simulink model "Hinf_sym1"  (R2023a)
settings: Solver=VariableStepAuto  StartTime=0.0  StopTime=500  RelTol=1e-3
InitFcn:
  | %Hinf_init
values from neighbouring files (symbols this model uses):
  C = [1 0 0 0; 0 1 0 0]    [Hinf_1DOF.m]    (also in Hinf_2DOFinit.m; Hinf_U_init.m; Hinf_WU_init.m; Hinf_init.m)
  dtheta_0 = 0    [Hinf_1DOF.m]    (also in Hinf_2DOFinit.m; Hinf_U_init.m; Hinf_WU_init.m; Hinf_init.m)
  dz_0 = 0    [Hinf_1DOF.m]    (also in Hinf_2DOFinit.m; Hinf_U_init.m; Hinf_WU_init.m; Hinf_init.m)
  fa_w = 0    [Hinf_1DOF.m]    (also in Hinf_2DOFinit.m; Hinf_U_init.m; Hinf_WU_init.m; Hinf_init.m)
  fm_w = s_param.g*s_param.m    [Hinf_1DOF.m]    (also in Hinf_2DOFinit.m; Hinf_U_init.m; Hinf_WU_init.m; Hinf_init.m)
  K = tf(ss(K.A,K.B,K.C,K.D))    [Hinf_U_init.m]    (also in Hinf_WU_init.m; Hinf_init.m)
  Km1 = 1.1    [Hinf_1DOF.m]    (also in Hinf_2DOFinit.m; Hinf_U_init.m; Hinf_WU_init.m; Hinf_init.m)
  Km1_real = Km1 + std_dev_Km*randn(1,1)    [Hinf_1DOF.m]    (also in Hinf_2DOFinit.m; Hinf_U_init.m; Hinf_WU_init.m; Hinf_init.m)
  Km2 = 1.1    [Hinf_1DOF.m]    (also in Hinf_2DOFinit.m; Hinf_U_init.m; Hinf_WU_init.m; Hinf_init.m)
  Km2_real = Km2 + std_dev_Km*randn(1,1)    [Hinf_1DOF.m]    (also in Hinf_2DOFinit.m; Hinf_U_init.m; Hinf_WU_init.m; Hinf_init.m)
  Kss = K    [Hinf_U_init.m]    (also in Hinf_WU_init.m; Hinf_init.m)
  out_rate = 0.001    [Hinf_1DOF.m]    (also in Hinf_2DOFinit.m; Hinf_U_init.m; Hinf_WU_init.m; Hinf_init.m)
  ss_global = ss(G)    [Hinf_init.m]
  T1 = 0.05    [Hinf_1DOF.m]    (also in Hinf_2DOFinit.m; Hinf_U_init.m; Hinf_WU_init.m; Hinf_init.m)
  T1_real = T1 + std_dev_T*randn(1,1)    [Hinf_1DOF.m]    (also in Hinf_2DOFinit.m; Hinf_U_init.m; Hinf_WU_init.m; Hinf_init.m)
  T2 = 0.15    [Hinf_1DOF.m]    (also in Hinf_2DOFinit.m; Hinf_U_init.m; Hinf_WU_init.m; Hinf_init.m)
  T2_real = T2 + std_dev_T*randn(1,1)    [Hinf_1DOF.m]    (also in Hinf_2DOFinit.m; Hinf_U_init.m; Hinf_WU_init.m; Hinf_init.m)
  theta_0_real = theta_0 + std_dev.theta_0*randn(1,1)    [Hinf_1DOF.m]    (also in Hinf_2DOFinit.m = theta_0+std_dev.theta_0*randn(1,1); Hinf_U_init.m = theta_0+std_dev.theta_0*randn(1,1); Hinf_WU_init.m = theta_0+std_dev.theta_0*randn(1,1); Hinf_init.m = theta_0+std_dev.theta_0*randn(1,1))
  theta_w = 0    [Hinf_1DOF.m]    (also in Hinf_2DOFinit.m; Hinf_U_init.m; Hinf_WU_init.m; Hinf_init.m)
  Tm1 = 1    [Hinf_1DOF.m]    (also in Hinf_2DOFinit.m; Hinf_U_init.m; Hinf_WU_init.m; Hinf_init.m)
  Tm1_real = Tm1 + std_dev_Tm*randn(1,1)    [Hinf_1DOF.m]    (also in Hinf_2DOFinit.m; Hinf_U_init.m; Hinf_WU_init.m; Hinf_init.m)
  Tm2 = 1    [Hinf_1DOF.m]    (also in Hinf_2DOFinit.m; Hinf_U_init.m; Hinf_WU_init.m; Hinf_init.m)
  Tm2_real = Tm2 + std_dev_Tm*randn(1,1)    [Hinf_1DOF.m]    (also in Hinf_2DOFinit.m; Hinf_U_init.m; Hinf_WU_init.m; Hinf_init.m)
  z_0_real = z_0 + std_dev.z_0*randn(1,1)    [Hinf_1DOF.m]    (also in Hinf_2DOFinit.m = z_0+std_dev.z_0*randn(1,1); Hinf_U_init.m = z_0+std_dev.z_0*randn(1,1); Hinf_WU_init.m = z_0+std_dev.z_0*randn(1,1); Hinf_init.m = z_0+std_dev.z_0*randn(1,1))
  z_w = 200    [Hinf_1DOF.m]    (also in Hinf_2DOFinit.m = 400; Hinf_U_init.m = 400; Hinf_WU_init.m = 400; Hinf_init.m = 400)
undefined symbols (not defined in the file or in its folder): s_param, s_param_r, std_dev
libraries: simulink x8
settings Model: Creator=franc  LastModifiedBy=franc

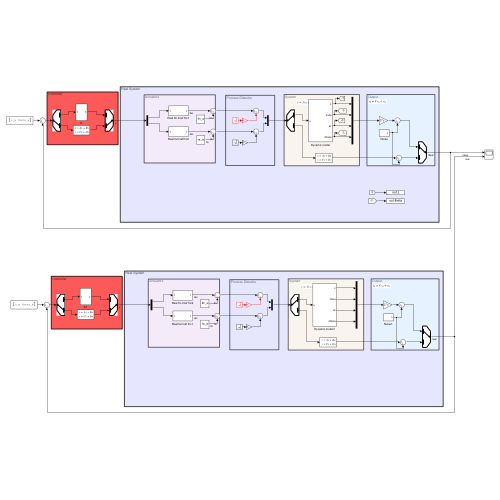
[thumbnail: Simulink's stored preview of the top-level diagram]
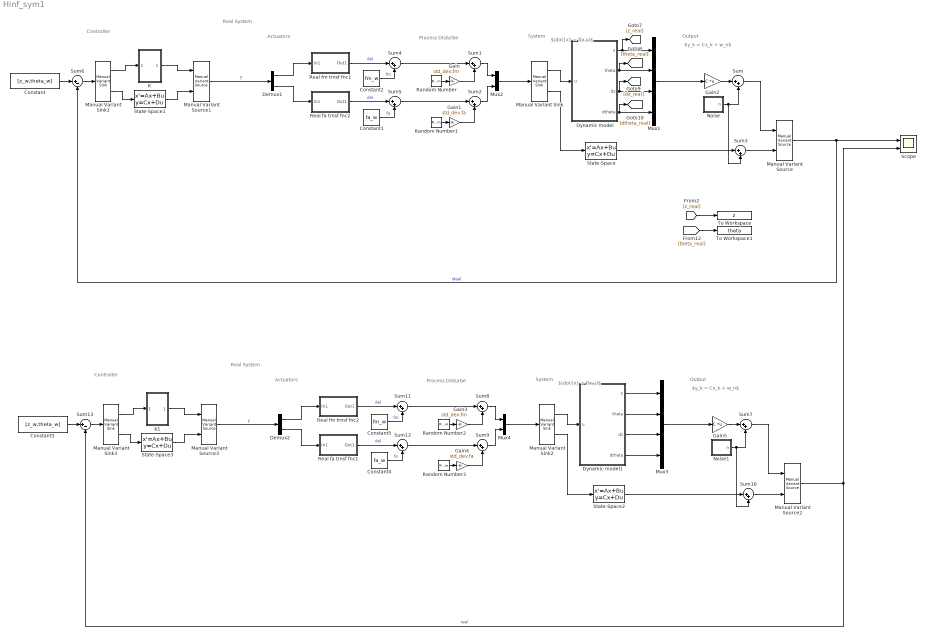
== system Hinf_sym1 ==
  note: Controller
  note: Real System
  note: Actuators
  note: Output
  note: $\dot{x} = f(x,u)$
  note: $y_k = Cx_k + w_n$
  note: System
  note: Process Disturbe
  note: Controller
  note: Real System
  note: Actuators
  note: Output
  note: $\dot{x} = f(x,u)$
  note: $y_k = Cx_k + w_n$
  note: System
  note: Process Disturbe
  Constant : Constant  Value=[z_w,theta_w]
  Constant1 : Constant  Value=fa_w
  Constant2 : Constant  Value=fm_w
  Constant3 : Constant  Value=[z_w,theta_w]
  Constant4 : Constant  Value=fa_w
  Constant5 : Constant  Value=fm_w
  Demux1 : Demux  Outputs=2
  Demux2 : Demux  Outputs=2
  Dynamic model : Subsystem
  Dynamic model1 : Subsystem
  Gain : Gain  Gain=std_dev.fm
  Gain1 : Gain  Gain=std_dev.fa
  Gain2 : Gain  Gain=C  Multiplication=Matrix(K*u)
  Gain3 : Gain  Gain=std_dev.fm
  Gain4 : Gain  Gain=std_dev.fa
  Gain5 : Gain  Gain=C  Multiplication=Matrix(K*u)
  K : Subsystem
  K1 : Subsystem
  Manual Variant Sink : simulink/Signal Routing/Manual Variant Sink  NumChoices=2  LabelModeActiveChoice=V_1
  Manual Variant Sink1 : simulink/Signal Routing/Manual Variant Sink  NumChoices=2  LabelModeActiveChoice=V_2
  Manual Variant Sink2 : simulink/Signal Routing/Manual Variant Sink  NumChoices=2  LabelModeActiveChoice=V_1
  Manual Variant Sink3 : simulink/Signal Routing/Manual Variant Sink  NumChoices=2  LabelModeActiveChoice=V_2
  Manual Variant Source : simulink/Signal Routing/Manual Variant Source  NumChoices=2  LabelModeActiveChoice=V_1
  Manual Variant Source1 : simulink/Signal Routing/Manual Variant Source  NumChoices=2  LabelModeActiveChoice=V_2
  Manual Variant Source2 : simulink/Signal Routing/Manual Variant Source  NumChoices=2  LabelModeActiveChoice=V_1
  Manual Variant Source3 : simulink/Signal Routing/Manual Variant Source  NumChoices=2  LabelModeActiveChoice=V_2
  Mux1 : Mux
  Mux2 : Mux  Inputs=2
  Mux3 : Mux
  Mux4 : Mux  Inputs=2
  Noise : Subsystem
  Noise1 : Subsystem
  Random Number{,1..3} (4 alike) : RandomNumber  SampleTime=out_rate
  Real fa trnsf fnc1 : Subsystem
  Real fa trnsf fnc2 : Subsystem
  Real fm trnsf fnc1 : Subsystem
  Real fm trnsf fnc2 : Subsystem
  Scope : Scope  NumInputPorts=2
  State-Space : StateSpace  A=ss_global.A  B=ss_global.B  C=ss_global.C  D=ss_global.D  InitialCondition=0
  State-Space1 : StateSpace  A=Kss.A  B=Kss.B  C=Kss.C  D=Kss.D  InitialCondition=0
  State-Space2 : StateSpace  A=ss_global.A  B=ss_global.B  C=ss_global.C  D=ss_global.D  InitialCondition=0
  State-Space3 : StateSpace  A=Kss.A  B=Kss.B  C=Kss.C  D=Kss.D  InitialCondition=0
  Sum{,1..5,7..12} (12 alike) : Sum  Inputs=|++
  Sum13 : Sum  Inputs=|+-
  Sum6 : Sum  Inputs=|+-
  To Workspace : ToWorkspace  VariableName=z  SaveFormat=Timeseries  SampleTime=-1
  To Workspace1 : ToWorkspace  VariableName=theta  SaveFormat=Timeseries  SampleTime=-1
  wires:
  Manual Variant Source/1 -> Scope/1, Sum6/2  "ideal"
  [theta_real] -> To Workspace1/1
  [z_real] -> To Workspace/1
  Random Number1/1 -> Gain1/1
  Random Number/1 -> Gain/1
  Gain/1 -> Sum1/2
  Manual Variant Sink/2 -> State-Space/1
  Real fa trnsf fnc2/1(Out1) -> Sum5/1  "del"
  Constant1/1 -> Sum5/2  "fa"
  Sum4/1 -> Sum1/1
  Sum/1 -> Manual Variant Source/1
  Mux1/1 -> Gain2/1
  State-Space/1 -> Sum3/1
  Sum1/1 -> Mux2/1
  Gain1/1 -> Sum2/2
  Sum3/1 -> Manual Variant Source/2
  Dynamic model/1(z) -> [z_real], Mux1/1
  Demux1/2 -> Real fa trnsf fnc2/1(In1)
  Noise/1(n) -> Sum/2, Sum3/2
  Dynamic model/3(dz) -> Mux1/3, [dz_real]
  Sum5/1 -> Sum2/1
  Dynamic model/2(theta) -> Mux1/2, [theta_real]
  Gain2/1 -> Sum/1
  Mux2/1 -> Manual Variant Sink/1
  Dynamic model/4(dtheta) -> Mux1/4, [dtheta_real]
  Sum2/1 -> Mux2/2
  Real fm trnsf fnc1/1(Out1) -> Sum4/1  "del"
  Demux1/1 -> Real fm trnsf fnc1/1(In1)
  Constant2/1 -> Sum4/2  "fm"
  Manual Variant Sink/1 -> Dynamic model/1(u)
  Sum6/1 -> Manual Variant Sink1/1
  K/1(Out1) -> Manual Variant Source1/1
  Constant/1 -> Sum6/1
  Manual Variant Source1/1 -> Demux1/1  "y"
  Manual Variant Sink1/1 -> K/1(In1)
  Manual Variant Sink1/2 -> State-Space1/1
  State-Space1/1 -> Manual Variant Source1/2
  State-Space3/1 -> Manual Variant Source3/2
  Manual Variant Sink3/2 -> State-Space3/1
  Manual Variant Sink3/1 -> K1/1(In1)
  Manual Variant Source3/1 -> Demux2/1  "y"
  Constant3/1 -> Sum13/1
  K1/1(Out1) -> Manual Variant Source3/1
  Sum13/1 -> Manual Variant Sink3/1
  Manual Variant Sink2/1 -> Dynamic model1/1(u)
  Constant5/1 -> Sum11/2  "fm"
  Demux2/1 -> Real fm trnsf fnc2/1(In1)
  Real fm trnsf fnc2/1(Out1) -> Sum11/1  "del"
  Sum9/1 -> Mux4/2
  Dynamic model1/4(dtheta) -> Mux3/4
  Mux4/1 -> Manual Variant Sink2/1
  Gain5/1 -> Sum7/1
  Dynamic model1/2(theta) -> Mux3/2
  Sum12/1 -> Sum9/1
  Dynamic model1/3(dz) -> Mux3/3
  Noise1/1(n) -> Sum10/2, Sum7/2
  Demux2/2 -> Real fa trnsf fnc1/1(In1)
  Dynamic model1/1(z) -> Mux3/1
  Sum10/1 -> Manual Variant Source2/2
  Gain4/1 -> Sum9/2
  Sum8/1 -> Mux4/1
  State-Space2/1 -> Sum10/1
  Mux3/1 -> Gain5/1
  Sum7/1 -> Manual Variant Source2/1
  Sum11/1 -> Sum8/1
  Constant4/1 -> Sum12/2  "fa"
  Real fa trnsf fnc1/1(Out1) -> Sum12/1  "del"
  Manual Variant Sink2/2 -> State-Space2/1
  Gain3/1 -> Sum8/2
  Random Number2/1 -> Gain3/1
  Random Number3/1 -> Gain4/1
  Manual Variant Source2/1 -> Scope/2, Sum13/2  "real"

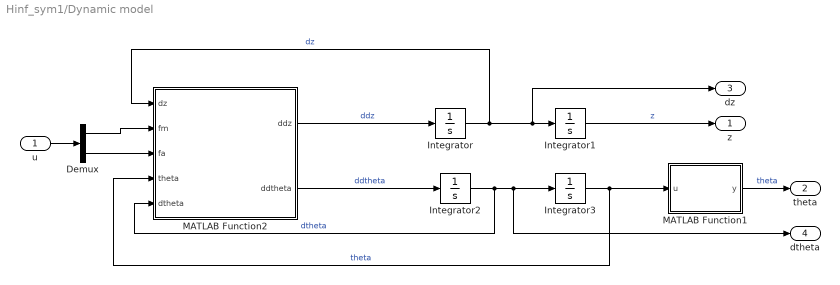
== system Hinf_sym1/Dynamic model ==
  u : Inport
  Demux : Demux  Outputs=2
  Integrator : Integrator  InitialCondition=dz_0
  Integrator1 : Integrator  InitialCondition=z_0_real
  Integrator2 : Integrator  InitialCondition=dtheta_0
  Integrator3 : Integrator  InitialCondition=theta_0_real
  MATLAB Function1 : MATLAB Function  TreatAsAtomicUnit=on
  MATLAB Function2 : MATLAB Function  TreatAsAtomicUnit=on
  z : Outport
  theta : Outport  Port=2
  dz : Outport  Port=3
  dtheta : Outport  Port=4
  wires:
  Integrator3/1 -> MATLAB Function2/4(theta), MATLAB Function1/1(u)  "theta"
  Integrator2/1 -> dtheta/1, Integrator3/1, MATLAB Function2/5(dtheta)  "dtheta"
  MATLAB Function1/1(y) -> theta/1  "theta"
  Integrator1/1 -> z/1  "z"
  MATLAB Function2/2(ddtheta) -> Integrator2/1  "ddtheta"
  MATLAB Function2/1(ddz) -> Integrator/1  "ddz"
  Integrator/1 -> dz/1, Integrator1/1, MATLAB Function2/1(dz)  "dz"
  u/1 -> Demux/1
  Demux/2 -> MATLAB Function2/3(fa)
  Demux/1 -> MATLAB Function2/2(fm)

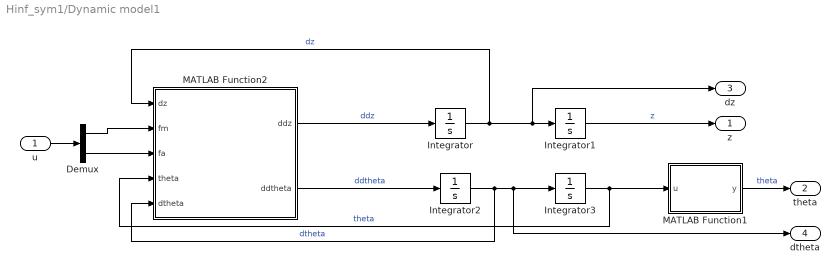
== system Hinf_sym1/Dynamic model1 ==
  u : Inport
  Demux : Demux  Outputs=2
  Integrator : Integrator  InitialCondition=dz_0
  Integrator1 : Integrator  InitialCondition=z_0_real
  Integrator2 : Integrator  InitialCondition=dtheta_0
  Integrator3 : Integrator  InitialCondition=theta_0_real
  MATLAB Function1 : MATLAB Function  TreatAsAtomicUnit=on
  MATLAB Function2 : MATLAB Function  TreatAsAtomicUnit=on
  z : Outport
  theta : Outport  Port=2
  dz : Outport  Port=3
  dtheta : Outport  Port=4
  wires:
  Demux/1 -> MATLAB Function2/2(fm)
  Demux/2 -> MATLAB Function2/3(fa)
  u/1 -> Demux/1
  Integrator/1 -> MATLAB Function2/1(dz), Integrator1/1, dz/1  "dz"
  MATLAB Function2/1(ddz) -> Integrator/1  "ddz"
  MATLAB Function2/2(ddtheta) -> Integrator2/1  "ddtheta"
  Integrator1/1 -> z/1  "z"
  MATLAB Function1/1(y) -> theta/1  "theta"
  Integrator2/1 -> MATLAB Function2/5(dtheta), Integrator3/1, dtheta/1  "dtheta"
  Integrator3/1 -> MATLAB Function1/1(u), MATLAB Function2/4(theta)  "theta"

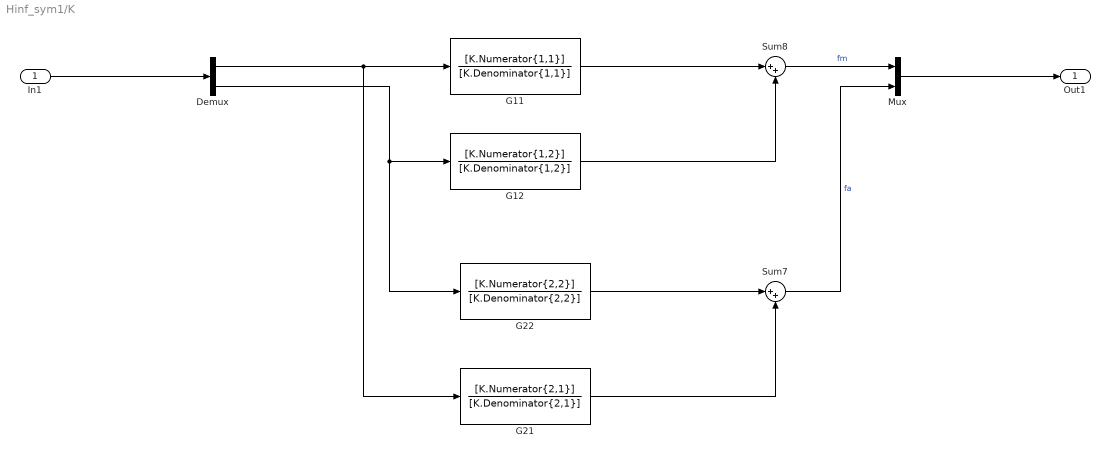
== system Hinf_sym1/K ==
  In1 : Inport
  Demux : Demux  Outputs=2
  G11 : TransferFcn  Numerator=[K.Numerator{1,1}]  Denominator=[K.Denominator{1,1}]
  G12 : TransferFcn  Numerator=[K.Numerator{1,2}]  Denominator=[K.Denominator{1,2}]
  G21 : TransferFcn  Numerator=[K.Numerator{2,1}]  Denominator=[K.Denominator{2,1}]
  G22 : TransferFcn  Numerator=[K.Numerator{2,2}]  Denominator=[K.Denominator{2,2}]
  Mux : Mux  Inputs=2
  Sum7 : Sum  Inputs=|++
  Sum8 : Sum  Inputs=|++
  Out1 : Outport
  wires:
  Sum7/1 -> Mux/2  "fa"
  Sum8/1 -> Mux/1  "fm"
  Demux/2 -> G22/1, G12/1
  G11/1 -> Sum8/1
  Demux/1 -> G21/1, G11/1
  G22/1 -> Sum7/1
  G12/1 -> Sum8/2
  G21/1 -> Sum7/2
  In1/1 -> Demux/1
  Mux/1 -> Out1/1

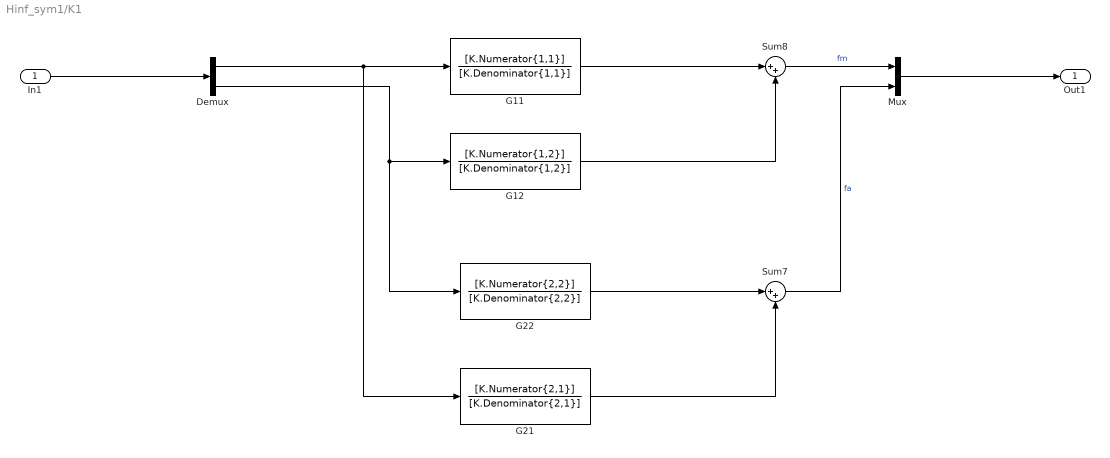
== system Hinf_sym1/K1 ==
  In1 : Inport
  Demux : Demux  Outputs=2
  G11 : TransferFcn  Numerator=[K.Numerator{1,1}]  Denominator=[K.Denominator{1,1}]
  G12 : TransferFcn  Numerator=[K.Numerator{1,2}]  Denominator=[K.Denominator{1,2}]
  G21 : TransferFcn  Numerator=[K.Numerator{2,1}]  Denominator=[K.Denominator{2,1}]
  G22 : TransferFcn  Numerator=[K.Numerator{2,2}]  Denominator=[K.Denominator{2,2}]
  Mux : Mux  Inputs=2
  Sum7 : Sum  Inputs=|++
  Sum8 : Sum  Inputs=|++
  Out1 : Outport
  wires:
  Mux/1 -> Out1/1
  In1/1 -> Demux/1
  G21/1 -> Sum7/2
  G12/1 -> Sum8/2
  G22/1 -> Sum7/1
  Demux/1 -> G11/1, G21/1
  G11/1 -> Sum8/1
  Demux/2 -> G12/1, G22/1
  Sum8/1 -> Mux/1  "fm"
  Sum7/1 -> Mux/2  "fa"

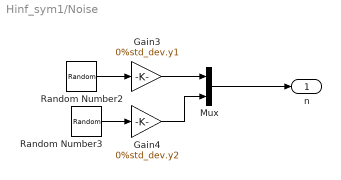
== system Hinf_sym1/Noise ==
  Gain3 : Gain  Gain=0%std_dev.y1
  Gain4 : Gain  Gain=0%std_dev.y2
  Mux : Mux  Inputs=2
  Random Number2 : RandomNumber  SampleTime=0.1
  Random Number3 : RandomNumber  SampleTime=0.1
  n : Outport
  wires:
  Random Number2/1 -> Gain3/1
  Random Number3/1 -> Gain4/1
  Gain4/1 -> Mux/2
  Mux/1 -> n/1
  Gain3/1 -> Mux/1

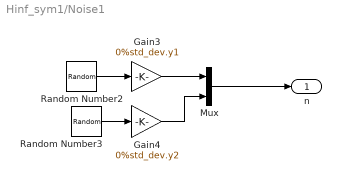
== system Hinf_sym1/Noise1 ==
  Gain3 : Gain  Gain=0%std_dev.y1
  Gain4 : Gain  Gain=0%std_dev.y2
  Mux : Mux  Inputs=2
  Random Number2 : RandomNumber  SampleTime=0.1
  Random Number3 : RandomNumber  SampleTime=0.1
  n : Outport
  wires:
  Gain3/1 -> Mux/1
  Mux/1 -> n/1
  Gain4/1 -> Mux/2
  Random Number3/1 -> Gain4/1
  Random Number2/1 -> Gain3/1

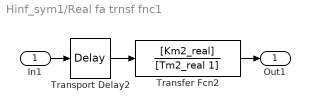
== system Hinf_sym1/Real fa trnsf fnc1 ==
  In1 : Inport
  Transfer Fcn2 : TransferFcn  Numerator=[Km2_real]  Denominator=[Tm2_real 1]
  Transport Delay2 : TransportDelay  DelayTime=T2_real
  Out1 : Outport
  wires:
  In1/1 -> Transport Delay2/1
  Transfer Fcn2/1 -> Out1/1
  Transport Delay2/1 -> Transfer Fcn2/1

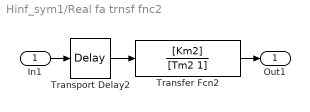
== system Hinf_sym1/Real fa trnsf fnc2 ==
  In1 : Inport
  Transfer Fcn2 : TransferFcn  Numerator=[Km2]  Denominator=[Tm2 1]
  Transport Delay2 : TransportDelay  DelayTime=T2
  Out1 : Outport
  wires:
  Transport Delay2/1 -> Transfer Fcn2/1
  Transfer Fcn2/1 -> Out1/1
  In1/1 -> Transport Delay2/1

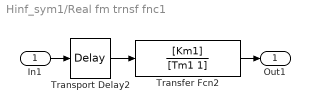
== system Hinf_sym1/Real fm trnsf fnc1 ==
  In1 : Inport
  Transfer Fcn2 : TransferFcn  Numerator=[Km1]  Denominator=[Tm1 1]
  Transport Delay2 : TransportDelay  DelayTime=T1
  Out1 : Outport
  wires:
  In1/1 -> Transport Delay2/1
  Transfer Fcn2/1 -> Out1/1
  Transport Delay2/1 -> Transfer Fcn2/1

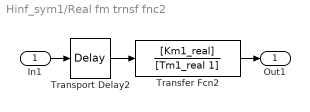
== system Hinf_sym1/Real fm trnsf fnc2 ==
  In1 : Inport
  Transfer Fcn2 : TransferFcn  Numerator=[Km1_real]  Denominator=[Tm1_real 1]
  Transport Delay2 : TransportDelay  DelayTime=T1_real
  Out1 : Outport
  wires:
  Transport Delay2/1 -> Transfer Fcn2/1
  Transfer Fcn2/1 -> Out1/1
  In1/1 -> Transport Delay2/1

== matlab function Hinf_sym1/Dynamic model1/MATLAB Function1 ==
  data: u input; y output
function y = fcn(u)

y = atan2(sin(u), cos(u));
end

== matlab function Hinf_sym1/Dynamic model/MATLAB Function2 ==
  data: dz input; fm input; fa input; ddz output; ddtheta output; theta input; dtheta input; s_param parameter
function [ddz, ddtheta] = fcn(dz, fm, fa, theta, dtheta, s_param)

% Rename params
J = s_param.J;     
m = s_param.m;     
b = s_param.b;      
beta = s_param.beta;    
g = s_param.g;     
l = s_param.l;   

%% Dynamic equations

ddz = -b/m * dz + fm/m * cos(theta) -g;
ddtheta = -beta/J * dtheta + 2 * l/J * fa;

end

== matlab function Hinf_sym1/Dynamic model1/MATLAB Function2 ==
  data: dz input; fm input; fa input; ddz output; ddtheta output; theta input; dtheta input; s_param_r parameter; s_param parameter
function [ddz, ddtheta] = fcn(dz, fm, fa, theta, dtheta,s_param_r, s_param)

% Rename params
J = s_param_r.J;     
m = s_param_r.m;     
b = s_param_r.b;      
beta = s_param_r.beta;    
g = s_param.g;     
l = s_param_r.l;   

%% Dynamic equations

ddz = -b/m * dz + fm/m * cos(theta) -g;
ddtheta = -beta/J * dtheta + 2 * l/J * fa;

end

== matlab function Hinf_sym1/Dynamic model/MATLAB Function1 ==
  data: u input; y output
function y = fcn(u)

y = atan2(sin(u), cos(u));
end
